simulink model "ComparaModeloTeorico"  (R2016a)
settings: Solver=VariableStepAuto  StartTime=0.0  StopTime=3000  RelTol=1e-3
values from neighbouring files (symbols this model uses):
  A = [a11 a12 a13 a14; a21 a22 a23 a24; a31 a32 a33 a34; a41 a42 a43 a44]    [RunMe.m]
  B = [b11 b12; b21 b22; b31 b32; b41 b42]    [RunMe.m]
  C = [0 0 1 0; 0 0 0 1]    [RunMe.m]
  D = [0 0; 0 0]    [RunMe.m]
libraries: realtime_pacer_lib x1
settings Model: Creator=tiago  LastModifiedBy=tiago

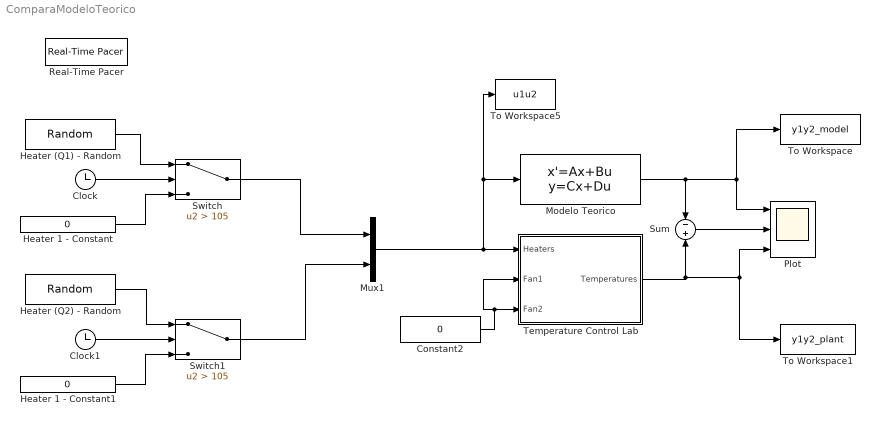
== system ComparaModeloTeorico ==
  Clock : Clock
  Clock1 : Clock
  Constant2 : Constant  Value=0
  Heater (Q1) - Random : RandomNumber  Mean=50  Variance=200  Seed=4  SampleTime=105
  Heater (Q2) - Random : RandomNumber  Mean=50  Variance=200  Seed=5  SampleTime=105
  Heater 1 - Constant : Constant  Value=0
  Heater 1 - Constant1 : Constant  Value=0
  Modelo Teorico : StateSpace  A=A  B=B  C=C  D=D  X0=0
  Mux1 : Mux  Inputs=2
  Plot : Scope  NumInputPorts=3
  Real-Time Pacer : realtime_pacer_lib/Real-Time Pacer  simTimePerRealTime=1
  Sum : Sum  Inputs=-|+
  Switch : Switch  Criteria=u2 > Threshold  Threshold=105
  Switch1 : Switch  Criteria=u2 > Threshold  Threshold=105
  Temperature Control Lab : Subsystem
      mask Display: image('tclab.png');
  To Workspace : ToWorkspace  VariableName=y1y2_model  SaveFormat=Timeseries  SampleTime=-1
  To Workspace1 : ToWorkspace  VariableName=y1y2_plant  SaveFormat=Timeseries  SampleTime=-1
  To Workspace5 : ToWorkspace  VariableName=u1u2  SaveFormat=Timeseries  SampleTime=-1
  wires:
  Mux1/1 -> To Workspace5/1, Modelo Teorico/1, Temperature Control Lab/1(Heaters)
  Constant2/1 -> Temperature Control Lab/2(Fan1), Temperature Control Lab/3(Fan2)
  Sum/1 -> Plot/2
  Modelo Teorico/1 -> To Workspace/1, Plot/1, Sum/1
  Temperature Control Lab/1(Temperatures) -> To Workspace1/1, Plot/3, Sum/2
  Heater (Q1) - Random/1 -> Switch/1
  Clock/1 -> Switch/2
  Heater 1 - Constant/1 -> Switch/3
  Heater (Q2) - Random/1 -> Switch1/1
  Clock1/1 -> Switch1/2
  Heater 1 - Constant1/1 -> Switch1/3
  Switch/1 -> Mux1/1
  Switch1/1 -> Mux1/2

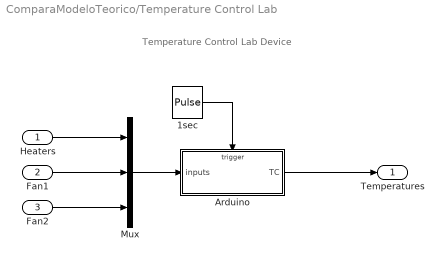
== system ComparaModeloTeorico/Temperature Control Lab ==
  note: Temperature Control Lab Device
  Heaters : Inport  PortDimensions=2
  Fan1 : Inport  Port=2  PortDimensions=1
  Fan2 : Inport  Port=3  PortDimensions=1
  1sec : DiscretePulseGenerator  PulseType=Time based  Period=0.5  PulseWidth=50
  Arduino : Subsystem  TreatAsAtomicUnit=on
  Mux : Mux  Inputs=3
  Temperatures : Outport
  wires:
  1sec/1 -> Arduino/Trigger
  Arduino/1(TC) -> Temperatures/1
  Mux/1 -> Arduino/1(inputs)
  Heaters/1 -> Mux/1
  Fan2/1 -> Mux/3
  Fan1/1 -> Mux/2

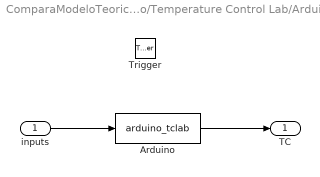
== system ComparaModeloTeorico/Temperature Control Lab/Arduino ==
  inputs : Inport  PortDimensions=4  LatchByDelayingOutsideSignal=on
  Trigger : TriggerPort  VariantControl=Variant
  Arduino : MATLABFcn  MATLABFcn=arduino_tclab
  TC : Outport  InitialOutput=[23 23]
  wires:
  inputs/1 -> Arduino/1
  Arduino/1 -> TC/1
